simulink model "sf_custom"  (Simulink 6.0)
settings: Solver=ode3  StartTime=0.0  StopTime=20  MaxStep=.1  RelTol=1e-3
settings Model: CovMetricSettings=dcmtr  Creator=The MathWorks Inc.  LastModifiedBy=batserve  ExtModeAutoUpdateStatusClock=off
settings DataIOCC: SignalLoggingName=sigsOut
settings OptimizationCC: BooleanDataType=off  InlineInvariantSignals=off  OptimizeModelRefInitCode=on  LifeSpan=1
settings DebuggingCC: CheckExecutionContextPreStartOutputMsg=on  CheckExecutionContextRuntimeOutputMsg=on  SolverPrmCheckMsg=none
settings HardwareCC: TargetHWDeviceType=32-bit Generic
settings RTWCC: SystemTargetFile=ert.tlc  TemplateMakefile=ert_default_tmf  Description=RTW Embedded Coder (no auto configuration)  ProcessScript=ert_make_rtw_hook  CustomSourceCode="#include \"my_header.h\""  CustomSource=my_function.c
settings CodeAppCC: IgnoreCustomStorageClasses=off
settings ERTTargetCC: TargetFcnLib=ansi_tfl_tmw.mat  GenFloatMathFcnCalls=ANSI_C  GenerateSampleERTMain=on  SupportContinuousTime=on  SupportNonInlinedSFcns=on  RootIOFormat=Individual Arguments  ERTCustomFileTemplate=example_file_process.tlc  InitialValueSource=Model

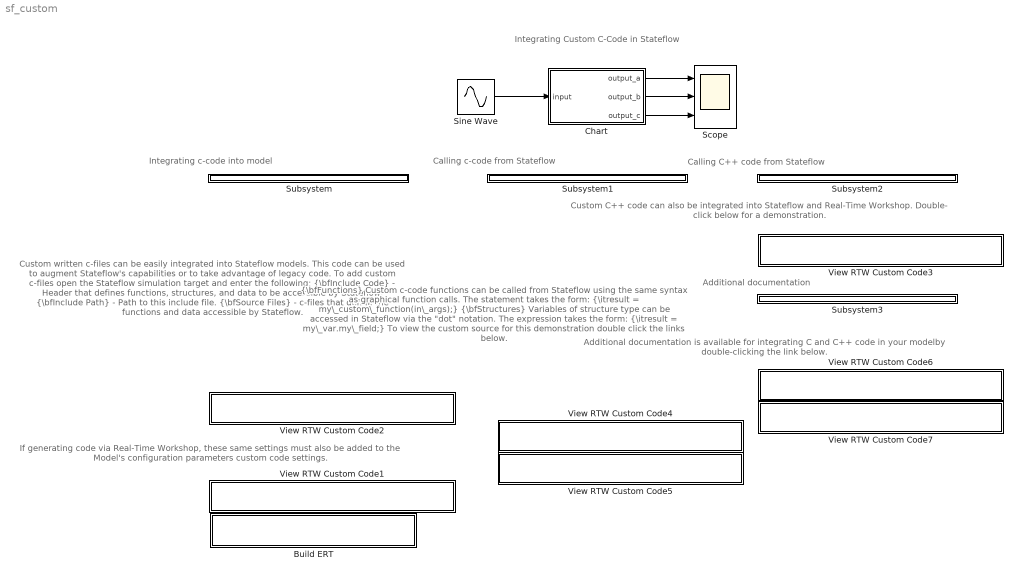
== system sf_custom ==
  note: Integrating Custom C-Code in Stateflow
  note: Calling C++ code from Stateflow
  note: Integrating c-code into model
  note: Calling c-code from Stateflow
  note: Custom written c-files can be easily integrated into
      | Stateflow models.  This code can be used to
      | augment Stateflow's capabilities or to take
      | advantage of legacy code.
      |
      | To add custom c-files open the Stateflow
      | simulation target and enter the following:
      |
      |   {\bfInclude Code} - Header that defines functions,
      |                               structures, and data to be
      |                               accessible by Stateflow.
      |   {\bfInclude Path} - Path to this include file.
      |   {\bfSource Files} - c-files that define the functions
      |                              and data accessible by Stateflow.
  note: If generating code via Real-Time Workshop, these
      | same settings must also be added to the Model's
      | configuration parameters custom code settings.
  note: {\bfFunctions}
      | Custom c-code functions can be called from
      | Stateflow using the same syntax as graphical
      | function calls.  The statement takes the form:
      |
      |   {\itresult = my\_custom\_function(in\_args);}
      |
      | {\bfStructures}
      | Variables of structure type can be accessed in
      | Stateflow via the "dot" notation.  The expression
      | takes the form:
      |
      |   {\itresult = my\_var.my\_field;}
      |
      | To view the custom source for this demonstration
      | double click the links below.
  note: Custom C++ code can also be integrated into
      | Stateflow and Real-Time Workshop.  Double-
      | click below for a demonstration.
  note: Additional documentation
  note: Additional documentation is available
      | for integrating C and C++ code in
      | your modelby double-clicking the link
      | below.
  Build ERT : Subsystem  PropExecContextAcrossSSBoundary=on  mask{attrib_overrides={}}
      mask prompts: attrib_overrides "List of attributes to preserve (cell of strings):"
      mask help: Enter the attributes of the configuration set that you want preserved. Otherwise, the default configuration script will override your current settings.
      mask init:
      | pos    = get_param(gcb, 'Position');
      | width  = pos(3) - pos(1);
      | height = pos(4) - pos(2);
      | 
      | 
      | % Compute arrow coordinates
      | arrowW = width  / 20;
      | arrowH = height / 2.5;
      | arrowX = width  / 50;
      | arrowY = height / 3;
      | arrowXvec = [arrowX, arrowX, arrowX + arrowW];
      | arrowYvec = [arrowY, arrowY + arrowH, arrowY + arrowH / 2];
      | 
      | % Compute text position
      | textXbuff = width / 30;
      | textX  = arrowX + arrowW + textXbuff;
      | textY  = height / 2;
      settings: OpenFcn=|
      | model=bdroot;
      | rtwbuilddemomodel(model);
      mask Display:
      | patch(arrowXvec, arrowYvec);
      | text(textX, textY, 'Build model using Real-Time\nWorkshop');
  Chart : Stateflow chart  PropExecContextAcrossSSBoundary=on
  Scope : Scope  NumInputPorts=3
      settings: TimeRange=20  YMin=-4~-2~1  YMax=4~2~3.5
  Sine Wave : Sin  SampleTime=0
  Subsystem : Subsystem  PropExecContextAcrossSSBoundary=on
  Subsystem1 : Subsystem  PropExecContextAcrossSSBoundary=on
  Subsystem2 : Subsystem  PropExecContextAcrossSSBoundary=on
  Subsystem3 : Subsystem  PropExecContextAcrossSSBoundary=on
  View RTW Custom Code1 : Subsystem  PropExecContextAcrossSSBoundary=on
      mask init: same as sf_custom/Build ERT
      settings: OpenFcn=|
      | slCfgPrmDlg(bdroot,'Open');
      | slCfgPrmDlg(bdroot,'TurnToPage','Real-Time Workshop/Symbols');
      mask Display:
      | patch(arrowXvec, arrowYvec);
      | text(textX, textY, 'Open Real-Time Workshop\ncustom code settings');
  View RTW Custom Code2 : Subsystem  PropExecContextAcrossSSBoundary=on
      mask init: same as sf_custom/Build ERT
      settings: OpenFcn=|
      | rt=sfroot;
      | m=rt.find('-isa','Stateflow.Machine','-and', 'name',bdroot);
      | tar=m.find('-isa','Stateflow.Target','-and','name','sfun');
      | sf('Private','targetddg_btn_target_cb',tar,'Target Options');
      mask Display:
      | patch(arrowXvec, arrowYvec);
      | text(textX, textY, 'Open Stateflow simulation\ncustom code settings');
  View RTW Custom Code3 : Subsystem  PropExecContextAcrossSSBoundary=on
      mask init: same as sf_custom/Build ERT
      settings: OpenFcn=sf_cpp
      mask Display:
      | patch(arrowXvec, arrowYvec);
      | text(textX, textY, 'Open sf_cpp');
  View RTW Custom Code4 : Subsystem  PropExecContextAcrossSSBoundary=on
      mask init: same as sf_custom/Build ERT
      settings: OpenFcn=eval('edit my_header.h')
      mask Display:
      | patch(arrowXvec, arrowYvec);
      | text(textX, textY, 'Open my_header.h');
  View RTW Custom Code5 : Subsystem  PropExecContextAcrossSSBoundary=on
      mask init: same as sf_custom/Build ERT
      settings: OpenFcn=eval('edit my_function.c')
      mask Display:
      | patch(arrowXvec, arrowYvec);
      | text(textX, textY, 'Open my_header.c');
  View RTW Custom Code6 : Subsystem  PropExecContextAcrossSSBoundary=on
      mask init: same as sf_custom/Build ERT
      settings: OpenFcn=helpview([docroot '/mapfiles/stateflow.map'], 'TARGET_OPTIONS_DIALOG')
      mask Display:
      | patch(arrowXvec, arrowYvec);
      | text(textX, textY, 'C-Code integration');
  View RTW Custom Code7 : Subsystem  PropExecContextAcrossSSBoundary=on
      mask init: same as sf_custom/Build ERT
      settings: OpenFcn=helpview([docroot '/mapfiles/stateflow.map'], 'including_custom_cpp_code')
      mask Display:
      | patch(arrowXvec, arrowYvec);
      | text(textX, textY, 'C++-Code integration');
  wires:
  Sine Wave/1 -> Chart/1(input)
  Chart/1(output_a) -> Scope/1
  Chart/2(output_b) -> Scope/2
  Chart/3(output_c) -> Scope/3

== system sf_custom/Build ERT ==

== system sf_custom/Subsystem ==

== system sf_custom/Subsystem1 ==

== system sf_custom/Subsystem2 ==

== system sf_custom/Subsystem3 ==

== system sf_custom/View RTW Custom Code1 ==

== system sf_custom/View RTW Custom Code2 ==

== system sf_custom/View RTW Custom Code3 ==

== system sf_custom/View RTW Custom Code4 ==

== system sf_custom/View RTW Custom Code5 ==

== system sf_custom/View RTW Custom Code6 ==

== system sf_custom/View RTW Custom Code7 ==

== stateflow chart Chart ==
  state One [parallel]
    state A
      during:
      gMyStructVar.a = input;
      output_a=gMyStructVar.a*3;
      output_b = my_function(input);
    (default) -> A
  state Two [parallel]
    state B
      during:
      gMyStructVar.b[1]=input+3;
      gMyStructPointerVar = &gMyStructVar;
      output_c=gMyStructPointerVar->b[1];
    (default) -> B
  note: In this demo, a C-code function defined in my_function.c and a structure that is defined
      | in my_header.h are included in the chart. MY_FUNCTION simply multiplies its input by
      | 2. The structure in my_header.h is defined as follows:
      | typedef struct {
      |                 real_T a;
      |                 int8_T b[10];
      | }MyStruct;
      | In the model, we access the structure member using the dot notation:  MyStruct.a and
      | also with the use of a pointer: gMyStructPointerVar ->b[1].  Notice that 'b' is defined as
      | an 8-bit integer value and not a Real (double) value. This the reason why 'output_c'
      | alternates between values '1' and '0' instead of taking the precise values of the input
      | sine wave.
  data: input input double size=1; output_a output double size=1; output_b output double size=1; output_c output double size=1
